simulink model "CCL_2"  (R2018a)
settings: Solver=ode4  StartTime=0  StopTime=inf  MaxStep=1e-4  RelTol=1e-3
InitFcn:
  | close
  | clear
  | clc
  | Sc=128
  | f=60;
  | T=1/f;
  | Ts=1/(f*Sc);
  | Vr=6500
  | V_v=[1    0.4    1          0.6       1       0.6       1       0.75   0.95]
  | T_v=[0   20/f  70/f    200/f   300/f     330/f   400/f   500/f  10]
  | S_time=60/f*20.5
  | V_R=3;
  | Tf=3
  | T_lc=3
  | set_param('CCL_2/EMISOR-RECEPTOR/TCP_IP_RX/ESCRITURA','Value','0')
undefined symbols (not defined in the file or in its folder): man, Vuc
libraries: simulink x3, libreria_comunicaciones_servidor2 x2, powerlib x1
settings Model: Creator=Mateo  LastModifiedBy=ana-n
settings CodeAppCC: StateflowObjectComments=on
settings SimscapeCC: SimscapeNormalizeSystem=off

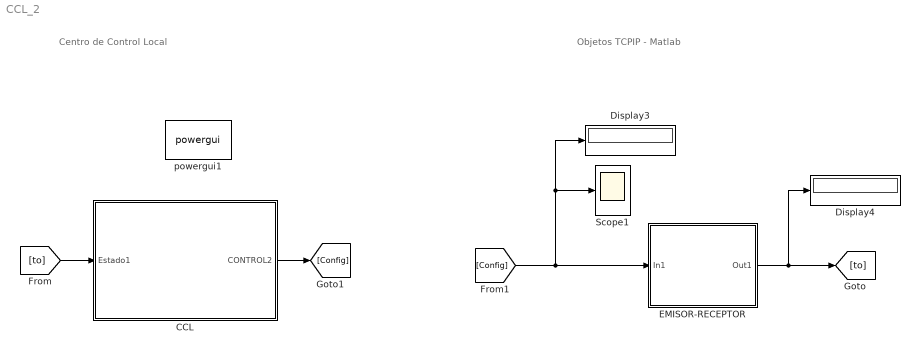
== system CCL_2 ==
  note: Centro de Control Local
  note: Objetos TCPIP - Matlab
  CCL : Subsystem  mask(Selector de etapa de operación del HAE){modo=Manual, manual=Etapa 2}
      mask help: Bloque del centro de control local con configuración manual y automática.
      mask TypeOptions modo: Automática | Manual
      mask Callback modo:
      | h1 = getSimulinkBlockHandle(gcb);
      | modo = get_param(h1,'modo');
      | if strcmp(modo,'Automática')
      |     Vuc=1;
      |     set_param(h1,'MaskVisibilities',{'on','off'});
      |     man=0;
      | elseif strcmp(modo,'Manual')
      |     Vuc=0;
      |     set_param(h1,'MaskVisibilities',{'on','on'});
      | end
      mask TypeOptions manual: Etapa 1 | Etapa 2 | Etapa 3
      mask Callback manual:
      | clc,
      | h2 = getSimulinkBlockHandle(gcb);
      | manuales = get_param(h2,'manual');
      | if strcmp(manuales,'Etapa 1')
      |     man=1;
      | elseif strcmp(manuales,'Etapa 2')
      |     man=2;
      | elseif strcmp(manuales,'Etapa 3')
      |     man=3;
      | end
      mask DialogControl ParameterGroupVar Prompt: Selección del tipo de configuración
      mask Display:
      | color('black');
      | disp('CCL');
      | %color('blue');
      | port_label('input',1,'Medida_t');
      | %color('red');
      | port_label('output',1,'Op_HAE');
  Display3 : Display
  Display4 : Display
  EMISOR-RECEPTOR : Subsystem
      mask Display:
      | port_label('output',1,'Receptor');
      | port_label('input',1,'Emisor');
  Scope1 : Scope
  powergui1 : powerlib/powergui  Priority=1  SimulationMode=Discrete  SampleTime=1/(60*128)  frequency=60  Iterations=50  frequencyindice=0  Pbase=100e6  ErrMax=1e-4  UnitsV=kV  UnitsW=MW  buscounter=0  FunctionMessages=off  echomessages=off  EnableUseOfTLC=off  CurrentSourceSwitches=on  DisableSnubberDevices=off  DisableRonSwitches=off  DisableVfSwitches=off  DisplayEquations=off  SolverType=Tustin/Backward Euler (TBE)  Interpol=off  ExternalGateDelay=off  methode=off  Ts=10  x0status=blocks  SPID=off  SwTol=0  HookPort=off  RestoreLinks=warning  ResistiveCurrentMeasurement=off  Frange=[0:2:500]  Ylog=off  Xlog=on  ShowGrid=off  save=off  variable=ZData  structure=0  ZoomFFT=off  StartTime=0.0  cycles=1  DisplayStyle=1  fundamental=60  FreqAxis=off  MaxFrequency=1000  frequencyindicesteady=1  RmsSteady=1  display=off
  wires:
  [to] -> CCL/1(Estado1)
  [Config] -> EMISOR-RECEPTOR/1(In1), Display3/1, Scope1/1
  CCL/1(CONTROL2) -> [Config]
  EMISOR-RECEPTOR/1(Out1) -> [to], Display4/1

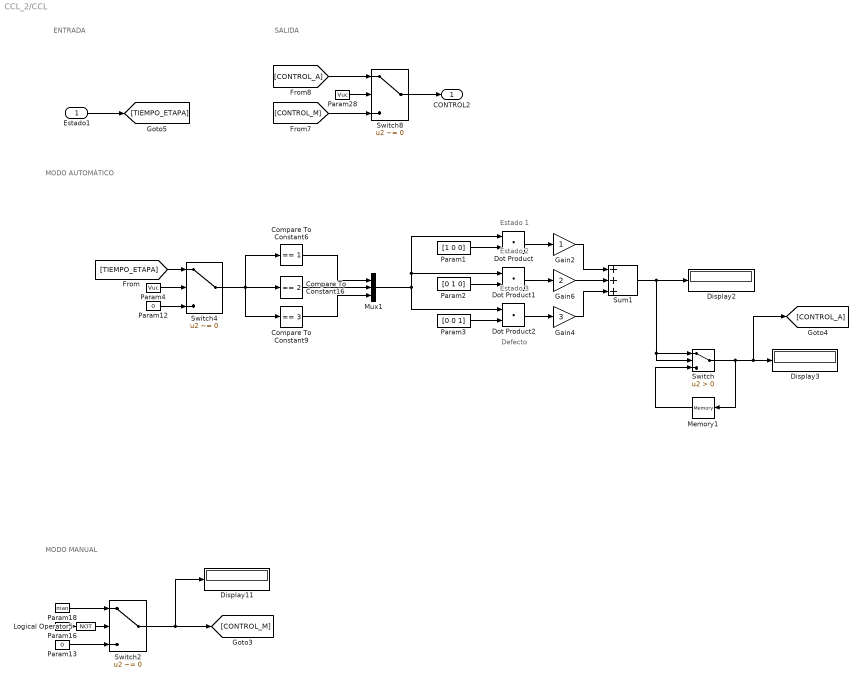
== system CCL_2/CCL ==
  note: Estado 3
  note: Defecto
  note: Estado 2
  note: Estado 1
  note: MODO MANUAL
  note: MODO AUTOMÁTICO
  note: SALIDA
  note: ENTRADA
  Estado1 : Inport
  Compare To Constant16 : simulink/Logic and Bit Operations/Compare To Constant  relop===  const=2  OutDataTypeStr=boolean
  Compare To Constant6 : simulink/Logic and Bit Operations/Compare To Constant  relop===  const=1  OutDataTypeStr=boolean
  Compare To Constant9 : simulink/Logic and Bit Operations/Compare To Constant  relop===  const=3  OutDataTypeStr=boolean
  Display11 : Display
  Display2 : Display
  Display3 : Display
  Dot Product : DotProduct  InputSameDT=on  OutDataTypeStr=Inherit: Inherit via internal rule
  Dot Product1 : DotProduct  InputSameDT=on  OutDataTypeStr=Inherit: Inherit via internal rule
  Dot Product2 : DotProduct  InputSameDT=on  OutDataTypeStr=Inherit: Inherit via internal rule
  Gain2 : Gain
  Gain4 : Gain  Gain=3
  Gain6 : Gain  Gain=2
  Logical Operator5 : Logic  Operator=NOT  AllPortsSameDT=off  OutDataTypeStr=boolean
  Memory1 : Memory  InitialCondition=1
  Mux1 : Mux  Inputs=3
  Param1 : Constant  Value=[1 0 0]  OutDataTypeStr=boolean
  Param12 : Constant  Value=0
  Param13 : Constant  Value=0
  Param16 : Constant  Value=Vuc
  Param18 : Constant  Value=man
  Param2 : Constant  Value=[0 1 0]  OutDataTypeStr=boolean
  Param28 : Constant  Value=Vuc
  Param3 : Constant  Value=[0 0 1]  OutDataTypeStr=boolean
  Param4 : Constant  Value=Vuc
  Sum1 : Sum  Inputs=+|+|+
  Switch : Switch  Criteria=u2 > Threshold  SaturateOnIntegerOverflow=on  InputSameDT=on
  Switch2 : Switch  Criteria=u2 ~= 0
  Switch4 : Switch  Criteria=u2 ~= 0
  Switch8 : Switch  Criteria=u2 ~= 0
  CONTROL2 : Outport
  wires:
  Compare To Constant9/1 -> Mux1/3
  Compare To Constant16/1 -> Mux1/2
  Compare To Constant6/1 -> Mux1/1
  Switch/1 -> Memory1/1, Display3/1, [CONTROL_A]
  Sum1/1 -> Display2/1, Switch/2, Switch/1
  Memory1/1 -> Switch/3
  Switch4/1 -> Compare To Constant16/1, Compare To Constant9/1, Compare To Constant6/1
  Param2/1 -> Dot Product1/2
  Param1/1 -> Dot Product/2
  Gain2/1 -> Sum1/1
  Dot Product1/1 -> Gain6/1
  Dot Product/1 -> Gain2/1
  Param3/1 -> Dot Product2/2
  Dot Product2/1 -> Gain4/1
  Mux1/1 -> Dot Product2/1, Dot Product1/1, Dot Product/1
  Gain4/1 -> Sum1/3
  Gain6/1 -> Sum1/2
  Estado1/1 -> [TIEMPO_ETAPA]
  Param4/1 -> Switch4/2
  Param12/1 -> Switch4/3
  [TIEMPO_ETAPA] -> Switch4/1
  Switch8/1 -> CONTROL2/1
  Param28/1 -> Switch8/2
  [CONTROL_M] -> Switch8/3
  [CONTROL_A] -> Switch8/1
  Switch2/1 -> Display11/1, [CONTROL_M]
  Param16/1 -> Logical Operator5/1
  Param13/1 -> Switch2/3
  Param18/1 -> Switch2/1
  Logical Operator5/1 -> Switch2/2

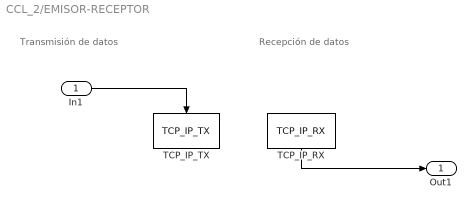
== system CCL_2/EMISOR-RECEPTOR ==
  note: Recepción de datos
  note: Transmisión de datos
  In1 : Inport
  TCP_IP_RX : libreria_comunicaciones_servidor2/TCP_IP_RX  SystemSampleTime=-1
      link override ESCRITURA: Value=server_1.dato_lectura
  TCP_IP_TX : libreria_comunicaciones_servidor2/TCP_IP_TX  SystemSampleTime=-1
  Out1 : Outport
  wires:
  TCP_IP_RX/1 -> Out1/1
  In1/1 -> TCP_IP_TX/1
